simulink model "Anti_Windup_Simu"  (R2020a)
settings: Solver=FixedStepAuto  StartTime=0.0  StopTime=100  FixedStep=0.05  RelTol=1e-3
values from neighbouring files (symbols this model uses):
  Kp = 1.85    [antiwindup.m]    (also in antiwindup_discreto.m)
  ti = 2.8    [antiwindup.m]    (also in antiwindup_discreto.m)
  tw = 1    [antiwindup_discreto.m]
  umax = 0.8    [antiwindup_discreto.m]
  umin = 0.0    (= 0)    [antiwindup_discreto.m]
libraries: cstblocks x2
settings Model: Creator=Sergio  LastModifiedBy=Sergio

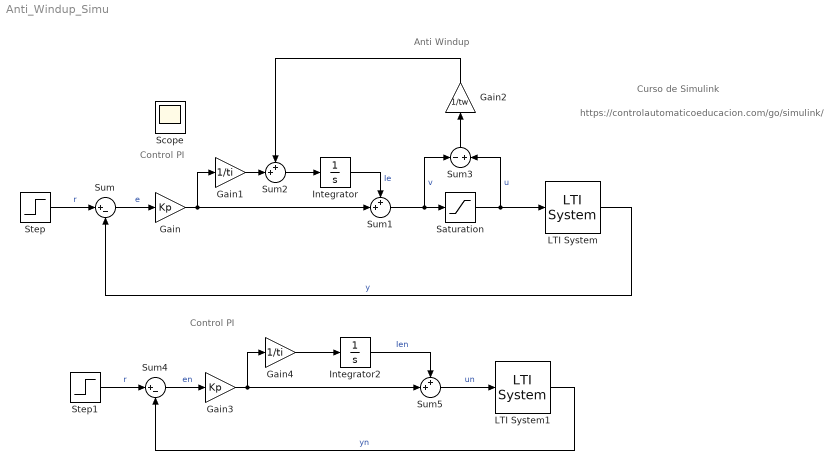
== system Anti_Windup_Simu ==
  note: https://controlautomaticoeducacion.com/go/simulink/
  note: Curso de Simulink
  note: Anti Windup
  note: Control PI
  note: Control PI
  Gain : Gain  Gain=Kp
  Gain1 : Gain  Gain=1/ti
  Gain2 : Gain  Gain=1/tw
  Gain3 : Gain  Gain=Kp
  Gain4 : Gain  Gain=1/ti
  Integrator : Integrator
  Integrator2 : Integrator
  LTI System : cstblocks/LTI System  sys=G  IC=[]
  LTI System1 : cstblocks/LTI System  sys=G  IC=[]
  Saturation : Saturate  UpperLimit=umax  LowerLimit=umin
  Step : Step  Time=10  After=0.5  SampleTime=0
  Step1 : Step  Time=10  After=0.5  SampleTime=0
  Sum : Sum  Inputs=|+-
  Sum1 : Sum  Inputs=++|
  Sum2 : Sum  Inputs=++|
  Sum3 : Sum  Inputs=-|+
  Sum4 : Sum  Inputs=|+-
  Sum5 : Sum  Inputs=++|
  Scope : Scope
  wires:
  Step/1 -> Sum/1  "r"
  LTI System/1 -> Sum/2  "y"
  Saturation/1 -> Sum3/2, LTI System/1  "u"
  Sum/1 -> Gain/1  "e"
  Gain/1 -> Sum1/2, Gain1/1
  Sum2/1 -> Integrator/1
  Sum1/1 -> Sum3/1, Saturation/1  "v"
  Sum3/1 -> Gain2/1
  Gain1/1 -> Sum2/2
  Gain2/1 -> Sum2/1
  Integrator/1 -> Sum1/1  "Ie"
  Integrator2/1 -> Sum5/1  "Ien"
  Sum5/1 -> LTI System1/1  "un"
  Gain4/1 -> Integrator2/1
  Gain3/1 -> Gain4/1, Sum5/2
  Sum4/1 -> Gain3/1  "en"
  LTI System1/1 -> Sum4/2  "yn"
  Step1/1 -> Sum4/1  "r"
